simulink model "3_Phase_Inverter"  (R2021a)
settings: Solver=VariableStepAuto  StartTime=0.0  StopTime=10.0  RelTol=1e-3
libraries: spsGtoLib x6, spsVoltageMeasurementLib x4, spsDCVoltageSourceLib x2, spsGroundLib x2, spspowerguiLib x1
settings Model: Creator=ritickgupta  LastModifiedBy=ritickgupta

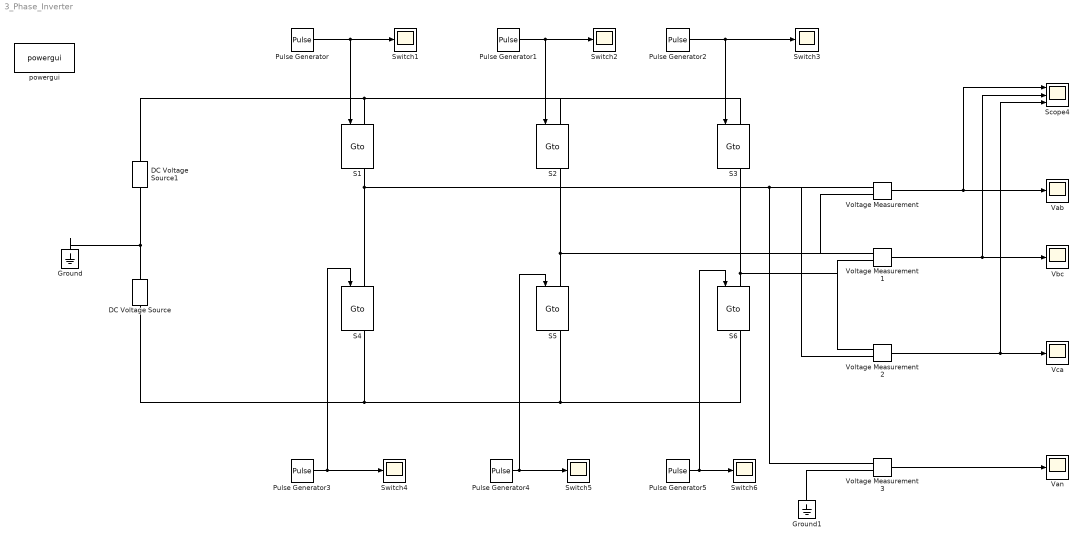
== system 3_Phase_Inverter ==
  DC Voltage Source : spsDCVoltageSourceLib/DC Voltage Source  Amplitude=100  Measurements=None
  DC Voltage Source1 : spsDCVoltageSourceLib/DC Voltage Source  Amplitude=100  Measurements=None
  Ground : spsGroundLib/Ground  LConnTagsString=a
  Ground1 : spsGroundLib/Ground  LConnTagsString=a
  Pulse Generator : DiscretePulseGenerator  PulseType=Time based  Period=3.6  PulseWidth=50
  Pulse Generator1 : DiscretePulseGenerator  PulseType=Time based  Period=3.6  PulseWidth=50  PhaseDelay=1.2
  Pulse Generator2 : DiscretePulseGenerator  PulseType=Time based  Period=3.6  PulseWidth=50  PhaseDelay=-1.2
  Pulse Generator3 : DiscretePulseGenerator  PulseType=Time based  Period=3.6  PulseWidth=50  PhaseDelay=1.8
  Pulse Generator4 : DiscretePulseGenerator  PulseType=Time based  Period=3.6  PulseWidth=50  PhaseDelay=-0.6
  Pulse Generator5 : DiscretePulseGenerator  PulseType=Time based  Period=3.6  PulseWidth=50  PhaseDelay=0.6
  S{1..6} (6 alike) : spsGtoLib/Gto  Ron=0.001  Lon=0  Vf=1  Tf=10e-6  Tt=20e-6  IC=0  Rs=1e5  Cs=inf  Measurements=on
      settings: SourceProductBaseCode=PS
  Scope4 : Scope  NumInputPorts=3
  Switch{1..6} (6 alike) : Scope
  Vab : Scope
  Van : Scope
  Vbc : Scope
  Vca : Scope
  Voltage Measurement{,1..3} (4 alike) : spsVoltageMeasurementLib/Voltage Measurement  PhasorSimulation=off  OutputType=Complex  PSBequivalent=0
  powergui : spspowerguiLib/powergui  Priority=1  SimulationMode=Continuous  SampleTime=50e-6  frequency=60  Iterations=50  frequencyindice=0  Pbase=100e6  ErrMax=1e-4  UnitsV=kV  UnitsW=MW  buscounter=0  FunctionMessages=off  echomessages=off  EnableUseOfTLC=off  CurrentSourceSwitches=off  DisableSnubberDevices=off  DisableRonSwitches=off  DisableVfSwitches=off  DisplayEquations=off  AutomaticDiscreteSolvers=off  SolverType=Tustin/Backward Euler (TBE)  Interpol=off  ExternalGateDelay=off  methode=off  Ts=100  x0status=blocks  SPID=on  SwTol=0  HookPort=off  NonlinearTolerance=1e-4  nMaxIteration=100  ContinueOnMaxIteration=off  RestoreLinks=warning  ResistiveCurrentMeasurement=off  Frange=[0:2:500]  Ylog=off  Xlog=on  ShowGrid=off  save=off  variable=ZData  structure=0  ZoomFFT=off  StartTime=0.0  cycles=1  DisplayStyle=1  fundamental=60  FreqAxis=off  MaxFrequency=1000  frequencyindicesteady=1  RmsSteady=1  display=off
  wires:
  Pulse Generator/1 -> Switch1/1, S1/1
  Pulse Generator1/1 -> Switch2/1, S2/1
  Pulse Generator2/1 -> Switch3/1, S3/1
  Pulse Generator3/1 -> Switch4/1, S4/1
  Pulse Generator4/1 -> Switch5/1, S5/1
  Pulse Generator5/1 -> Switch6/1, S6/1
  Voltage Measurement/1 -> Scope4/1, Vab/1
  Voltage Measurement1/1 -> Scope4/2, Vbc/1
  Voltage Measurement2/1 -> Scope4/3, Vca/1
  Voltage Measurement3/1 -> Van/1
  connections:
  DC Voltage Source1/RConn1 -- S3/LConn1 -- S2/LConn1 -- S1/LConn1
  S3/RConn1 -- Voltage Measurement1/LConn2 -- Voltage Measurement2/LConn1 -- S6/LConn1
  S6/RConn1 -- S5/RConn1 -- S4/RConn1 -- DC Voltage Source/LConn1
  DC Voltage Source1/LConn1 -- Ground/LConn1 -- DC Voltage Source/RConn1
  S1/RConn1 -- Voltage Measurement3/LConn1 -- Voltage Measurement2/LConn2 -- Voltage Measurement/LConn1 -- S4/LConn1
  S2/RConn1 -- Voltage Measurement/LConn2 -- Voltage Measurement1/LConn1 -- S5/LConn1
  Ground1/LConn1 -- Voltage Measurement3/LConn2
